simulink model "RCAM_Sim_TrimTest"  (R2020a)
settings: Solver=VariableStepAuto  StartTime=0.0  StopTime=TF  RelTol=1e-3
values from neighbouring files (symbols this model uses):
  u1max = 25*(pi/180)    (= 0.436332312999)    [ValidateTrimPoint.m]    (also in initSim.m)
  u1min = -25*(pi/180)    (= -0.436332312999)    [ValidateTrimPoint.m]    (also in initSim.m)
  u2max = 10*(pi/180)    (= 0.174532925199)    [ValidateTrimPoint.m]    (also in initSim.m)
  u2min = -25*(pi/180)    (= -0.436332312999)    [ValidateTrimPoint.m]    (also in initSim.m)
  u3max = 30*(pi/180)    (= 0.523598775598)    [ValidateTrimPoint.m]    (also in initSim.m)
  u3min = -30*(pi/180)    (= -0.523598775598)    [ValidateTrimPoint.m]    (also in initSim.m)
  u4max = 10*(pi/180)    (= 0.174532925199)    [ValidateTrimPoint.m]    (also in initSim.m)
  u4min = 0    [ValidateTrimPoint.m]    (also in initSim.m)
  u5max = 10*(pi/180)    (= 0.174532925199)    [ValidateTrimPoint.m]    (also in initSim.m)
  u5min = 0.5*(pi/180)    (= 0.00872664625997)    [ValidateTrimPoint.m]    (also in initSim.m)
  UStar = ZStar(10:14)    [TrimRCAM.m]    (also in ValidateTrimPoint.m = temp.UStar; trim_values_sl.mat = [4.57898508613e-08 -0.178007605555 1.17251054893e-07 0.08208)
  XStar = ZStar(1:9)    [TrimRCAM.m]    (also in ValidateTrimPoint.m = temp.XStar; trim_values_sl.mat = [84.990492012 1.83039692313e-09 1.27132479689 -4.0525614012e)
settings Model: Creator=brian  LastModifiedBy=brian

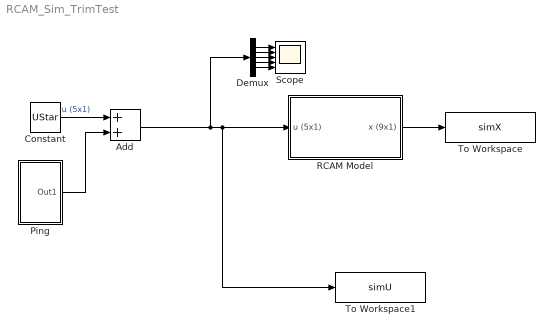
== system RCAM_Sim_TrimTest ==
  Add : Sum
  Constant : Constant  Value=UStar
  Demux : Demux  Outputs=5
  Ping : Subsystem
  RCAM Model : Subsystem
  Scope : Scope  NumInputPorts=5
  To Workspace : ToWorkspace  VariableName=simX  SaveFormat=Timeseries  SampleTime=-1
  To Workspace1 : ToWorkspace  VariableName=simU  SaveFormat=Timeseries  SampleTime=-1
  wires:
  RCAM Model/1(x (9x1)) -> To Workspace/1
  Demux/1 -> Scope/1
  Demux/2 -> Scope/2
  Demux/3 -> Scope/3
  Demux/4 -> Scope/4
  Demux/5 -> Scope/5
  Constant/1 -> Add/1  "u (5x1)"
  Ping/1(Out1) -> Add/2
  Add/1 -> Demux/1, To Workspace1/1, RCAM Model/1(u (5x1))

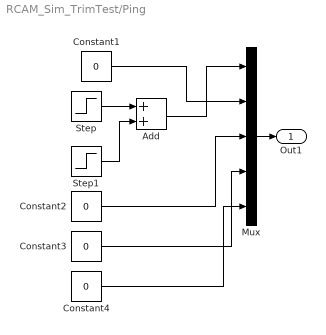
== system RCAM_Sim_TrimTest/Ping ==
  Add : Sum
  Constant{1..4} (4 alike) : Constant  Value=0
  Mux : Mux  Inputs=5
  Step : Step  Time=5  After=5*pi/180  SampleTime=0
  Step1 : Step  Time=7  After=-5*pi/180  SampleTime=0
  Out1 : Outport
  wires:
  Constant4/1 -> Mux/5
  Constant2/1 -> Mux/3
  Mux/1 -> Out1/1
  Constant3/1 -> Mux/4
  Step/1 -> Add/1
  Step1/1 -> Add/2
  Add/1 -> Mux/1
  Constant1/1 -> Mux/2

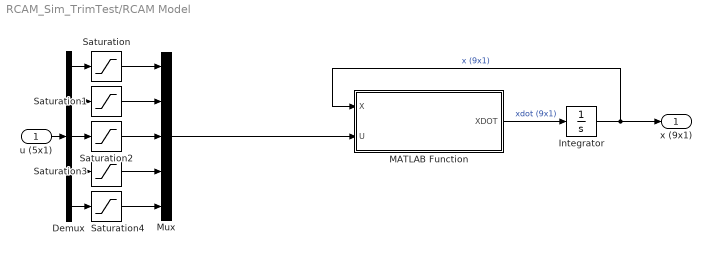
== system RCAM_Sim_TrimTest/RCAM Model ==
  u (5x1) : Inport
  Demux : Demux  Outputs=5
  Integrator : Integrator  InitialCondition=XStar
  MATLAB Function : MATLAB Function  TreatAsAtomicUnit=on
  Mux : Mux  Inputs=5
  Saturation : Saturate  UpperLimit=u1max  LowerLimit=u1min
  Saturation1 : Saturate  UpperLimit=u2max  LowerLimit=u2min
  Saturation2 : Saturate  UpperLimit=u3max  LowerLimit=u3min
  Saturation3 : Saturate  UpperLimit=u4max  LowerLimit=u4min
  Saturation4 : Saturate  UpperLimit=u5max  LowerLimit=u5min
  x (9x1) : Outport
  wires:
  MATLAB Function/1(XDOT) -> Integrator/1  "xdot (9x1)"
  Integrator/1 -> x (9x1)/1, MATLAB Function/1(X)  "x (9x1)"
  u (5x1)/1 -> Demux/1
  Demux/1 -> Saturation/1
  Demux/2 -> Saturation1/1
  Demux/3 -> Saturation2/1
  Demux/4 -> Saturation3/1
  Demux/5 -> Saturation4/1
  Saturation/1 -> Mux/1
  Saturation1/1 -> Mux/2
  Saturation2/1 -> Mux/3
  Saturation3/1 -> Mux/4
  Saturation4/1 -> Mux/5
  Mux/1 -> MATLAB Function/2(U)

== matlab function RCAM_Sim_TrimTest/RCAM Model/MATLAB Function ==
  data: X input; XDOT output; U input
function XDOT    = RCAM_model_wrapper(X, U)

[XDOT] = RCAM_model(X, U);
